simulink model "MAS_FTESO"  (R2022b)
settings: Solver=ode4  StartTime=0.0  StopTime=30  FixedStep=0.01  RelTol=1e-3
(part 2 of 3)

== matlab function MAS_FTESO/Control and plant 5/LP-based controller/Linear programming optimisation ==
  data: u_nom input; u_i output; G_i input; now output; expect output; expect input
function [u_i, now, expect] = linear_programming(u_nom, G_i, expect)

%% This function performs the optimisation via linear programming
% Input:
% u_ei: The nominal sliding mode control input for error reduction
% u_mi: The nominal sliding mode control input for acceleration tracking
% G_i: The control gain matrix
% Output:
% u_i: The optimised control input
% expect: The expected control performance

%% Find out the constrains
U_M = 0.2;

% Saturate the maintain control input
% u_mi_max = U_M;
% u_mi = min( u_mi_max * ones(size(u_mi)) , max(u_mi , - u_mi_max * ones(size(u_mi))) );

flag = 0;
u_i = u_nom;
for i = 1 : size(u_i,1)
    if abs(u_i(i))>U_M
        flag = 1;   % flag turns 1 if the limit is reached
        break;
    end
end

% Call the linear programming solver from MATLAB
coder.extrinsic('linprog');

if flag == 1
    
    %% Intialisation
    % Restrictions on inequalities
    A_ine = zeros(2*size(u_nom,1), size(u_nom,1));
    b_ine = zeros(2*size(u_nom,1), 1);
    num_ine = 0;
    
    % Restrictions on qualities
    A_equ = zeros(2*size(u_nom,1), size(u_nom,1));
    b_equ = zeros(2*size(u_nom,1), 1);
    num_equ = 0;
    
    %% Upper and lower bound from saturation
    lb = - U_M * ones(size(u_nom));
    ub = U_M * ones(size(u_nom));
    
    %% Restrictions according to expect
    for i = 1 : size(u_nom,1)
        if expect(i) == 0 % leading to equalities
            num_equ = num_equ + 1;
            A_equ(num_equ, :) = G_i(i,:);
        else
            % No extra effort
            num_ine = num_ine + 1;
            A_ine(num_ine,:) = sign(expect(i)) * G_i(i,:);
            b_ine(num_ine) = abs(expect(i));
            
            % Avoid inverse effect (same sign)
            num_ine = num_ine + 1;
            A_ine(num_ine,:) = - sign(expect(i)) * G_i(i,:);
            
        end
    end
    
    %% Restriction to keep the same direction   
       
    % Average cost function
    F_4 = -G_i(1,:) * sign(expect(1)) - G_i(2,:) * sign(expect(2)) - G_i(3,:) * sign(expect(3));
    
    F_5 = -G_i(1,:) * expect(1) - G_i(2,:) * expect(2) - G_i(3,:) * expect(3);
    
    F=F_4;

    u_i = linprog(F,A_ine(1:num_ine,:),b_ine(1:num_ine), A_equ(1:num_equ,:), b_equ(1:num_equ),lb,ub);
end

now = G_i * u_i;

end

== matlab function MAS_FTESO/Control and plant 4/Information subtracting ==
  data: e_xi output; L input; info_commu input; info_control input; delta_xi output; delta_vi output; a_di output; u_i_hat output; s_i output
function [e_xi, delta_xi, delta_vi, a_di, u_i_hat, s_i]=info_subtracting(L, info_commu,info_control)

%% This function is built to subtract the useful information for the controller design

% info_commu is in the format of [x_1,v_1,....,x_N,v_N]
% info_control is in the format of [delta_xi, delta_vi, a_di, w_i_hat]

serial_num = 4;
dimension = 3;
lambda = 2;

% For multiple system, we first seperate info_commu into delta_xi and delta_vi
num_agent = size(L,1);

delta_x = kron( kron(eye(num_agent) , [1,0] ), eye(dimension) ) * info_commu;
delta_v = kron( kron(eye(num_agent) , [0,1] ), eye(dimension) ) * info_commu;

L_i = kron( L(serial_num,:), eye(dimension) );
    
% Local errors calculating
e_xi = L_i * delta_x;
e_vi = L_i * delta_v;

% Substracting info_control
delta_xi = info_control(dimension*0+1:dimension*1);
delta_vi = info_control(dimension*1+1:dimension*2);

a_di = info_control(dimension*2+1:dimension*3);
u_i_hat = info_control(dimension*3+1:dimension*4);

% Slide variable
s_i = lambda * e_xi + e_vi;

end

== matlab function MAS_FTESO/Control and plant 4/LP-based controller/Linear programming optimisation ==
  data: u_nom input; u_i output; G_i input; now output; expect output; expect input
function [u_i, now, expect] = linear_programming(u_nom, G_i, expect)

%% This function performs the optimisation via linear programming
% Input:
% u_ei: The nominal sliding mode control input for error reduction
% u_mi: The nominal sliding mode control input for acceleration tracking
% G_i: The control gain matrix
% Output:
% u_i: The optimised control input
% expect: The expected control performance

%% Find out the constrains
U_M = 0.2;

% Saturate the maintain control input
% u_mi_max = U_M;
% u_mi = min( u_mi_max * ones(size(u_mi)) , max(u_mi , - u_mi_max * ones(size(u_mi))) );

flag = 0;
u_i = u_nom;
for i = 1 : size(u_i,1)
    if abs(u_i(i))>U_M
        flag = 1;   % flag turns 1 if the limit is reached
        break;
    end
end

% Call the linear programming solver from MATLAB
coder.extrinsic('linprog');

if flag == 1
    
    %% Intialisation
    % Restrictions on inequalities
    A_ine = zeros(2*size(u_nom,1), size(u_nom,1));
    b_ine = zeros(2*size(u_nom,1), 1);
    num_ine = 0;
    
    % Restrictions on qualities
    A_equ = zeros(2*size(u_nom,1), size(u_nom,1));
    b_equ = zeros(2*size(u_nom,1), 1);
    num_equ = 0;
    
    %% Upper and lower bound from saturation
    lb = - U_M * ones(size(u_nom));
    ub = U_M * ones(size(u_nom));
    
    %% Restrictions according to expect
    for i = 1 : size(u_nom,1)
        if expect(i) == 0 % leading to equalities
            num_equ = num_equ + 1;
            A_equ(num_equ, :) = G_i(i,:);
        else
            % No extra effort
            num_ine = num_ine + 1;
            A_ine(num_ine,:) = sign(expect(i)) * G_i(i,:);
            b_ine(num_ine) = abs(expect(i));
            
            % Avoid inverse effect (same sign)
            num_ine = num_ine + 1;
            A_ine(num_ine,:) = - sign(expect(i)) * G_i(i,:);
            
        end
    end
    
    %% Restriction to keep the same direction   
       
    % Average cost function
    F_4 = -G_i(1,:) * sign(expect(1)) - G_i(2,:) * sign(expect(2)) - G_i(3,:) * sign(expect(3));
    
    F_5 = -G_i(1,:) * expect(1) - G_i(2,:) * expect(2) - G_i(3,:) * expect(3);
    
    F=F_4;

    u_i = linprog(F,A_ine(1:num_ine,:),b_ine(1:num_ine), A_equ(1:num_equ,:), b_equ(1:num_equ),lb,ub);
end

now = G_i * u_i;

end

== matlab function MAS_FTESO/Control and plant 3/Information subtracting ==
  data: e_xi output; L input; info_commu input; info_control input; delta_xi output; delta_vi output; a_di output; u_i_hat output; s_i output
function [e_xi, delta_xi, delta_vi, a_di, u_i_hat, s_i]=info_subtracting(L, info_commu,info_control)

%% This function is built to subtract the useful information for the controller design

% info_commu is in the format of [x_1,v_1,....,x_N,v_N]
% info_control is in the format of [delta_xi, delta_vi, a_di, w_i_hat]

serial_num = 3;
dimension = 3;
lambda = 2;

% For multiple system, we first seperate info_commu into delta_xi and delta_vi
num_agent = size(L,1);

delta_x = kron( kron(eye(num_agent) , [1,0] ), eye(dimension) ) * info_commu;
delta_v = kron( kron(eye(num_agent) , [0,1] ), eye(dimension) ) * info_commu;

L_i = kron( L(serial_num,:), eye(dimension) );
    
% Local errors calculating
e_xi = L_i * delta_x;
e_vi = L_i * delta_v;

% Substracting info_control
delta_xi = info_control(dimension*0+1:dimension*1);
delta_vi = info_control(dimension*1+1:dimension*2);

a_di = info_control(dimension*2+1:dimension*3);
u_i_hat = info_control(dimension*3+1:dimension*4);

% Slide variable
s_i = lambda * e_xi + e_vi;

end

== matlab function MAS_FTESO/Self-calculation 3/Observer/Estimation sliding surface ==
  data: state input; state_hat input; esti_x output
function esti_x   = esti_slide(state,state_hat)

%% This function represents the self-iteration of the observer itself
dimension = 3;

% Seperate the state information
x = state(dimension*0+1:dimension*1);

% Seperate the state estiamtion
x_hat = state_hat(dimension*0+1:dimension*1);

% Estimation error vectors
esti_x = x - x_hat;

end

== matlab function MAS_FTESO/Control and plant 3/LP-based controller/Linear programming optimisation ==
  data: u_nom input; u_i output; G_i input; now output; expect output; expect input
function [u_i, now, expect] = linear_programming(u_nom, G_i, expect)

%% This function performs the optimisation via linear programming
% Input:
% u_ei: The nominal sliding mode control input for error reduction
% u_mi: The nominal sliding mode control input for acceleration tracking
% G_i: The control gain matrix
% Output:
% u_i: The optimised control input
% expect: The expected control performance

%% Find out the constrains
U_M = 0.2;

% Saturate the maintain control input
% u_mi_max = U_M;
% u_mi = min( u_mi_max * ones(size(u_mi)) , max(u_mi , - u_mi_max * ones(size(u_mi))) );

flag = 0;
u_i = u_nom;
for i = 1 : size(u_i,1)
    if abs(u_i(i))>U_M
        flag = 1;   % flag turns 1 if the limit is reached
        break;
    end
end

% Call the linear programming solver from MATLAB
coder.extrinsic('linprog');

if flag == 1
    
    %% Intialisation
    % Restrictions on inequalities
    A_ine = zeros(2*size(u_nom,1), size(u_nom,1));
    b_ine = zeros(2*size(u_nom,1), 1);
    num_ine = 0;
    
    % Restrictions on qualities
    A_equ = zeros(2*size(u_nom,1), size(u_nom,1));
    b_equ = zeros(2*size(u_nom,1), 1);
    num_equ = 0;
    
    %% Upper and lower bound from saturation
    lb = - U_M * ones(size(u_nom));
    ub = U_M * ones(size(u_nom));
    
    %% Restrictions according to expect
    for i = 1 : size(u_nom,1)
        if expect(i) == 0 % leading to equalities
            num_equ = num_equ + 1;
            A_equ(num_equ, :) = G_i(i,:);
        else
            % No extra effort
            num_ine = num_ine + 1;
            A_ine(num_ine,:) = sign(expect(i)) * G_i(i,:);
            b_ine(num_ine) = abs(expect(i));
            
            % Avoid inverse effect (same sign)
            num_ine = num_ine + 1;
            A_ine(num_ine,:) = - sign(expect(i)) * G_i(i,:);
            
        end
    end
    
    %% Restriction to keep the same direction   
       
    % Average cost function
    F_4 = -G_i(1,:) * sign(expect(1)) - G_i(2,:) * sign(expect(2)) - G_i(3,:) * sign(expect(3));
    
    F_5 = -G_i(1,:) * expect(1) - G_i(2,:) * expect(2) - G_i(3,:) * expect(3);
    
    F=F_4;

    u_i = linprog(F,A_ine(1:num_ine,:),b_ine(1:num_ine), A_equ(1:num_equ,:), b_equ(1:num_equ),lb,ub);
end

now = G_i * u_i;

end

== matlab function MAS_FTESO/Control and plant 1/LP-based controller/Nominal Controller ==
  data: x_i input; u_i output; delta_xi input; delta_vi input; a_di input; u_i_hat input; s_i input; xi_i input; G_i output; expect output
function [u_i, G_i, expect] = fcn(x_i, delta_xi, delta_vi, a_di, u_i_hat, s_i, xi_i)

%% This is the controller design for each agent
%% Controller parameters
c_i = 2;
lambda_i = 2;

%% Basic model parameters
Radius = [0.20,0.22,0.21,0.19,0.23,0.18];   

%% The parameter of individual agent
serial_num = 1; 
R=Radius(serial_num);

%% Robot orientation
theta = x_i(3);

%% Input coupling matrix
G_i=[-sin(theta), -sin(pi/3-theta), sin(pi/3+theta);
    cos(theta), -cos(pi/3-theta), -cos(pi/3+theta);
    1/R,          1/R,                  1/R];

%% Nominal control input
expect = a_di - u_i_hat - lambda_i * delta_vi - c_i * s_i - delta_xi - c_i * xi_i;
u_i = G_i^(-1) * expect;

end

== matlab function MAS_FTESO/Control and plant 3/LP-based controller/Nominal Controller ==
  data: x_i input; u_i output; delta_xi input; delta_vi input; a_di input; u_i_hat input; s_i input; xi_i input; G_i output; expect output
function [u_i, G_i, expect] = fcn(x_i, delta_xi, delta_vi, a_di, u_i_hat, s_i, xi_i)

%% This is the controller design for each agent
%% Controller parameters
c_i = 2;
lambda_i = 2;

%% Basic model parameters
Radius = [0.20,0.22,0.21,0.19,0.23,0.18];   

%% The parameter of individual agent
serial_num = 3; 
R=Radius(serial_num);

%% Robot orientation
theta = x_i(3);

%% Input coupling matrix
G_i=[-sin(theta), -sin(pi/3-theta), sin(pi/3+theta);
    cos(theta), -cos(pi/3-theta), -cos(pi/3+theta);
    1/R,          1/R,                  1/R];

%% Nominal control input
expect = a_di - u_i_hat - lambda_i * delta_vi - c_i * s_i - delta_xi - c_i * xi_i;
u_i = G_i^(-1) * expect;

end

== matlab function MAS_FTESO/Self-calculation 1/Observer/Estimation sliding surface ==
  data: state input; state_hat input; esti_x output
function esti_x   = esti_slide(state,state_hat)

%% This function represents the self-iteration of the observer itself
dimension = 3;

% Seperate the state information
x = state(dimension*0+1:dimension*1);

% Seperate the state estiamtion
x_hat = state_hat(dimension*0+1:dimension*1);

% Estimation error vectors
esti_x = x - x_hat;

end

== matlab function MAS_FTESO/Self-calculation 1/Observer/MATLAB Function ==
  data: state_hat input; w_i_hat output
function w_i_hat = fcn(state_hat)

dimension = 3;

w_i_hat = state_hat(dimension * 2 + 1 : dimension * 3);

end

== matlab function MAS_FTESO/Self-calculation 2/Observer/Estimation sliding surface ==
  data: state input; state_hat input; esti_x output
function esti_x   = esti_slide(state,state_hat)

%% This function represents the self-iteration of the observer itself
dimension = 3;

% Seperate the state information
x = state(dimension*0+1:dimension*1);

% Seperate the state estiamtion
x_hat = state_hat(dimension*0+1:dimension*1);

% Estimation error vectors
esti_x = x - x_hat;

end

== matlab function MAS_FTESO/Self-calculation 2/Observer/MATLAB Function ==
  data: state_hat input; w_i_hat output
function w_i_hat = fcn(state_hat)

dimension = 3;

w_i_hat = state_hat(dimension * 2 + 1 : dimension * 3);

end

== matlab function MAS_FTESO/Self-calculation 1/Observer/Observer iteration ==
  data: state_hat_dot output; state input; u_i input; x_tilde input; state_hat input
function state_hat_dot  = eso(state, u_i, x_tilde, state_hat)

serial_num = 1;
dimension = 3;
Radius = [0.20,0.22,0.21,0.19,0.23,0.18];
R = Radius(serial_num);
theta = state(dimension);
g=[-sin(theta), -sin(pi/3-theta), sin(pi/3+theta);
    cos(theta), -cos(pi/3-theta), -cos(pi/3+theta);
    1/R,          1/R,                  1/R];

alpha_1 = 4/5;
alpha_2 = 3/5;
beta_1 = 5 * eye(3);
beta_2 = 10 * eye(3);
beta_3 = 100 * eye(3);
rho = 2 * eye(3);

x_hat_dot = state_hat(dimension * 1 + 1 : dimension * 2) + beta_1 * (diag(sign(x_tilde)) * abs(x_tilde).^alpha_1 + x_tilde );
v_hat_dot = state_hat(dimension * 2 + 1 : dimension * 3) + beta_2 * (diag(sign(x_tilde)) * abs(x_tilde).^alpha_2 + rho * x_tilde ) + g * u_i;
w_hat_dot = beta_3 * ( diag(sign(x_tilde)) * abs(x_tilde).^alpha_2 + rho * x_tilde );

state_hat_dot = [x_hat_dot; v_hat_dot; w_hat_dot]; 

end

== matlab function MAS_FTESO/Self-calculation 3/Observer/MATLAB Function ==
  data: state_hat input; w_i_hat output
function w_i_hat = fcn(state_hat)

dimension = 3;

w_i_hat = state_hat(dimension * 2 + 1 : dimension * 3);

end

== matlab function MAS_FTESO/Control and plant 1/System Plant1 ==
  settings: updateMethod=DISCRETE
  data: agent_x input; v_dot output; agent_v input; t input; control_input input; w output
function [v_dot, w] = physical_model( agent_x , agent_v, t, control_input )

%% Note
% System output
% v_dot: the acceleration vector
% w: the matched disturbances
% saturation status: off
% model is established by the driving force provided by the motor

%% basic parameters set of agents
Mass = [3,3.2,2.8,2.6,3.1,2.9];
Radius = [0.20,0.22,0.21,0.19,0.23,0.18];
Inertia = [0.08,0.10,0.07,0.05,0.09,0.06];

%% assign the parameter according to serial number
serial_num = 1; 
m=Mass(serial_num);
R=Radius(serial_num);
inertia=Inertia(serial_num);

%% current states of the robot
dimension=3;

x=agent_x(1);
y=agent_x(2);
theta=agent_x(dimension);

%% time-varying matched disturbances
% matched_disturbance= [0.5*sin(1.5*t+pi/4*serial_num+x)+2; 0.6*cos(2*t+pi/3*serial_num+0.5*y)+1.5; 0.5*sin(0.8*t+pi/5*serial_num+0.4*theta)+1];

% matched_disturbance= [0.5*sin(1.5*t+pi/4*serial_num)+2; 0.6*cos(2*t+pi/3*serial_num)+1.5; 0.5*sin(0.8*t+pi/5*serial_num)+1];
matched_disturbance = 0.2 * [0.5*sin(x) + 0.5*sin(0.6*t + pi/5*serial_num); - 0.6*exp(-abs(y)-1) + 0.4*sin(0.4*t + pi/5*serial_num) ; 0.2 * cos(theta) + 0.3 * sin(0.5*t + pi/5*serial_num)];
% matched_disturbance = matched_disturbance + noise;
%% the real model of robot
M=diag([1/m,1/m,1/inertia]);
g=[-sin(theta), -sin(pi/3-theta), sin(pi/3+theta);
    cos(theta), -cos(pi/3-theta), -cos(pi/3+theta);
    1/R,          1/R,                  1/R];


%% plant output

w = matched_disturbance;

v_dot = w + g* control_input;


end

== matlab function MAS_FTESO/Control and plant 4/LP-based controller/Nominal Controller ==
  data: x_i input; u_i output; delta_xi input; delta_vi input; a_di input; u_i_hat input; s_i input; xi_i input; G_i output; expect output
function [u_i, G_i, expect] = fcn(x_i, delta_xi, delta_vi, a_di, u_i_hat, s_i, xi_i)

%% This is the controller design for each agent
%% Controller parameters
c_i = 2;
lambda_i = 2;

%% Basic model parameters
Radius = [0.20,0.22,0.21,0.19,0.23,0.18];   

%% The parameter of individual agent
serial_num = 4; 
R=Radius(serial_num);

%% Robot orientation
theta = x_i(3);

%% Input coupling matrix
G_i=[-sin(theta), -sin(pi/3-theta), sin(pi/3+theta);
    cos(theta), -cos(pi/3-theta), -cos(pi/3+theta);
    1/R,          1/R,                  1/R];

%% Nominal control input
expect = a_di - u_i_hat - lambda_i * delta_vi - c_i * s_i - delta_xi - c_i * xi_i;
u_i = G_i^(-1) * expect;

end

== matlab function MAS_FTESO/Control and plant 5/LP-based controller/Nominal Controller ==
  data: x_i input; u_i output; delta_xi input; delta_vi input; a_di input; u_i_hat input; s_i input; xi_i input; G_i output; expect output
function [u_i, G_i, expect] = fcn(x_i, delta_xi, delta_vi, a_di, u_i_hat, s_i, xi_i)

%% This is the controller design for each agent
%% Controller parameters
c_i = 2;
lambda_i = 2;

%% Basic model parameters
Radius = [0.20,0.22,0.21,0.19,0.23,0.18];   

%% The parameter of individual agent
serial_num = 5; 
R=Radius(serial_num);

%% Robot orientation
theta = x_i(3);

%% Input coupling matrix
G_i=[-sin(theta), -sin(pi/3-theta), sin(pi/3+theta);
    cos(theta), -cos(pi/3-theta), -cos(pi/3+theta);
    1/R,          1/R,                  1/R];

%% Nominal control input
expect = a_di - u_i_hat - lambda_i * delta_vi - c_i * s_i - delta_xi - c_i * xi_i;
u_i = G_i^(-1) * expect;

end

== matlab function MAS_FTESO/Control and plant 6/LP-based controller/Nominal Controller ==
  data: x_i input; u_i output; delta_xi input; delta_vi input; a_di input; u_i_hat input; s_i input; xi_i input; G_i output; expect output
function [u_i, G_i, expect] = fcn(x_i, delta_xi, delta_vi, a_di, u_i_hat, s_i, xi_i)

%% This is the controller design for each agent
%% Controller parameters
c_i = 2;
lambda_i = 2;

%% Basic model parameters
Radius = [0.20,0.22,0.21,0.19,0.23,0.18];   

%% The parameter of individual agent
serial_num = 6; 
R=Radius(serial_num);

%% Robot orientation
theta = x_i(3);

%% Input coupling matrix
G_i=[-sin(theta), -sin(pi/3-theta), sin(pi/3+theta);
    cos(theta), -cos(pi/3-theta), -cos(pi/3+theta);
    1/R,          1/R,                  1/R];

%% Nominal control input
expect = a_di - u_i_hat - lambda_i * delta_vi - c_i * s_i - delta_xi - c_i * xi_i;
u_i = G_i^(-1) * expect;

end

== matlab function MAS_FTESO/Control and plant 1/LP-based controller/Subsystem/Auxiliary variable ==
  data: G_i input; u_tilde input; xi_dot output; xi_prev input
function xi_dot = aux_updata(G_i, u_tilde, xi_prev)

eta_4 = diag([3,3,2]);
eta_5 = diag([0.5,0.5,0.5]);

if norm(xi_prev) >= 10
    xi_dot = eta_4 * G_i * u_tilde - eta_5 * xi_prev;
else
    xi_dot = eta_4 * G_i * u_tilde - eta_5 * xi_prev - norm(u_tilde)^2/norm(xi_prev)^2 * xi_prev;
end

end

== matlab function MAS_FTESO/Self-calculation 4/Observer/Estimation sliding surface ==
  data: state input; state_hat input; esti_x output
function esti_x   = esti_slide(state,state_hat)

%% This function represents the self-iteration of the observer itself
dimension = 3;

% Seperate the state information
x = state(dimension*0+1:dimension*1);

% Seperate the state estiamtion
x_hat = state_hat(dimension*0+1:dimension*1);

% Estimation error vectors
esti_x = x - x_hat;

end

== matlab function MAS_FTESO/Self-calculation 3/Observer/Observer iteration ==
  data: state_hat_dot output; state input; u_i input; x_tilde input; state_hat input
function state_hat_dot  = eso(state, u_i, x_tilde, state_hat)

serial_num = 3;
dimension = 3;
Radius = [0.20,0.22,0.21,0.19,0.23,0.18];
R = Radius(serial_num);
theta = state(dimension);
g=[-sin(theta), -sin(pi/3-theta), sin(pi/3+theta);
    cos(theta), -cos(pi/3-theta), -cos(pi/3+theta);
    1/R,          1/R,                  1/R];

alpha_1 = 4/5;
alpha_2 = 3/5;
beta_1 = 5 * eye(3);
beta_2 = 10 * eye(3);
beta_3 = 100 * eye(3);
rho = 2 * eye(3);

x_hat_dot = state_hat(dimension * 1 + 1 : dimension * 2) + beta_1 * (diag(sign(x_tilde)) * abs(x_tilde).^alpha_1 + x_tilde );
v_hat_dot = state_hat(dimension * 2 + 1 : dimension * 3) + beta_2 * (diag(sign(x_tilde)) * abs(x_tilde).^alpha_2 + rho * x_tilde ) + g * u_i;
w_hat_dot = beta_3 * ( diag(sign(x_tilde)) * abs(x_tilde).^alpha_2 + rho * x_tilde );

state_hat_dot = [x_hat_dot; v_hat_dot; w_hat_dot]; 

end

== matlab function MAS_FTESO/Self-calculation 4/Observer/MATLAB Function ==
  data: state_hat input; w_i_hat output
function w_i_hat = fcn(state_hat)

dimension = 3;

w_i_hat = state_hat(dimension * 2 + 1 : dimension * 3);

end

== matlab function MAS_FTESO/Control and plant 3/LP-based controller/Subsystem/Auxiliary variable ==
  data: G_i input; u_tilde input; xi_dot output; xi_prev input
function xi_dot = aux_updata(G_i, u_tilde, xi_prev)

eta_4 = diag([3,3,2]);
eta_5 = diag([0.5,0.5,0.5]);

if norm(xi_prev) >= 10
    xi_dot = eta_4 * G_i * u_tilde - eta_5 * xi_prev;
else
    xi_dot = eta_4 * G_i * u_tilde - eta_5 * xi_prev - norm(u_tilde)^2/norm(xi_prev)^2 * xi_prev;
end

end

== matlab function MAS_FTESO/Self-calculation 4/Observer/Observer iteration ==
  data: state_hat_dot output; state input; u_i input; x_tilde input; state_hat input
function state_hat_dot  = eso(state, u_i, x_tilde, state_hat)

serial_num = 4;
dimension = 3;
Radius = [0.20,0.22,0.21,0.19,0.23,0.18];
R = Radius(serial_num);
theta = state(dimension);
g=[-sin(theta), -sin(pi/3-theta), sin(pi/3+theta);
    cos(theta), -cos(pi/3-theta), -cos(pi/3+theta);
    1/R,          1/R,                  1/R];

alpha_1 = 4/5;
alpha_2 = 3/5;
beta_1 = 5 * eye(3);
beta_2 = 10 * eye(3);
beta_3 = 100 * eye(3);
rho = 2 * eye(3);

x_hat_dot = state_hat(dimension * 1 + 1 : dimension * 2) + beta_1 * (diag(sign(x_tilde)) * abs(x_tilde).^alpha_1 + x_tilde );
v_hat_dot = state_hat(dimension * 2 + 1 : dimension * 3) + beta_2 * (diag(sign(x_tilde)) * abs(x_tilde).^alpha_2 + rho * x_tilde ) + g * u_i;
w_hat_dot = beta_3 * ( diag(sign(x_tilde)) * abs(x_tilde).^alpha_2 + rho * x_tilde );

state_hat_dot = [x_hat_dot; v_hat_dot; w_hat_dot]; 

end

== matlab function MAS_FTESO/Control and plant 4/LP-based controller/Subsystem/Auxiliary variable ==
  data: G_i input; u_tilde input; xi_dot output; xi_prev input
function xi_dot = aux_updata(G_i, u_tilde, xi_prev)

eta_4 = diag([3,3,2]);
eta_5 = diag([0.5,0.5,0.5]);

if norm(xi_prev) >= 10
    xi_dot = eta_4 * G_i * u_tilde - eta_5 * xi_prev;
else
    xi_dot = eta_4 * G_i * u_tilde - eta_5 * xi_prev - norm(u_tilde)^2/norm(xi_prev)^2 * xi_prev;
end

end

== matlab function MAS_FTESO/Control and plant 5/LP-based controller/Subsystem/Auxiliary variable ==
  data: G_i input; u_tilde input; xi_dot output; xi_prev input
function xi_dot = aux_updata(G_i, u_tilde, xi_prev)

eta_4 = diag([3,3,2]);
eta_5 = diag([0.5,0.5,0.5]);

if norm(xi_prev) >= 10
    xi_dot = eta_4 * G_i * u_tilde - eta_5 * xi_prev;
else
    xi_dot = eta_4 * G_i * u_tilde - eta_5 * xi_prev - norm(u_tilde)^2/norm(xi_prev)^2 * xi_prev;
end

end

== matlab function MAS_FTESO/Control and plant 6/LP-based controller/Subsystem/Auxiliary variable ==
  data: G_i input; u_tilde input; xi_dot output; xi_prev input
function xi_dot = aux_updata(G_i, u_tilde, xi_prev)

eta_4 = diag([3,3,2]);
eta_5 = diag([0.5,0.5,0.5]);

if norm(xi_prev) >= 10
    xi_dot = eta_4 * G_i * u_tilde - eta_5 * xi_prev;
else
    xi_dot = eta_4 * G_i * u_tilde - eta_5 * xi_prev - norm(u_tilde)^2/norm(xi_prev)^2 * xi_prev;
end

end

== matlab function MAS_FTESO/Self-calculation 5/Observer1/Estimation sliding surface ==
  data: state input; state_hat input; esti_x output
function esti_x   = esti_slide(state,state_hat)

%% This function represents the self-iteration of the observer itself
dimension = 3;

% Seperate the state information
x = state(dimension*0+1:dimension*1);

% Seperate the state estiamtion
x_hat = state_hat(dimension*0+1:dimension*1);

% Estimation error vectors
esti_x = x - x_hat;

end

== matlab function MAS_FTESO/Self-calculation 5/Observer1/MATLAB Function ==
  data: state_hat input; w_i_hat output
function w_i_hat = fcn(state_hat)

dimension = 3;

w_i_hat = state_hat(dimension * 2 + 1 : dimension * 3);

end

== matlab function MAS_FTESO/Self-calculation 5/Observer1/Observer iteration ==
  data: state_hat_dot output; state input; u_i input; x_tilde input; state_hat input
function state_hat_dot  = eso(state, u_i, x_tilde, state_hat)

serial_num = 5;
dimension = 3;
Radius = [0.20,0.22,0.21,0.19,0.23,0.18];
R = Radius(serial_num);
theta = state(dimension);
g=[-sin(theta), -sin(pi/3-theta), sin(pi/3+theta);
    cos(theta), -cos(pi/3-theta), -cos(pi/3+theta);
    1/R,          1/R,                  1/R];

alpha_1 = 4/5;
alpha_2 = 3/5;
beta_1 = 5 * eye(3);
beta_2 = 10 * eye(3);
beta_3 = 100 * eye(3);
rho = 2 * eye(3);

x_hat_dot = state_hat(dimension * 1 + 1 : dimension * 2) + beta_1 * (diag(sign(x_tilde)) * abs(x_tilde).^alpha_1 + x_tilde );
v_hat_dot = state_hat(dimension * 2 + 1 : dimension * 3) + beta_2 * (diag(sign(x_tilde)) * abs(x_tilde).^alpha_2 + rho * x_tilde ) + g * u_i;
w_hat_dot = beta_3 * ( diag(sign(x_tilde)) * abs(x_tilde).^alpha_2 + rho * x_tilde );

state_hat_dot = [x_hat_dot; v_hat_dot; w_hat_dot]; 

end

== matlab function MAS_FTESO/Self-calculation 6/Observer1/Estimation sliding surface ==
  data: state input; state_hat input; esti_x output
function esti_x   = esti_slide(state,state_hat)

%% This function represents the self-iteration of the observer itself
dimension = 3;

% Seperate the state information
x = state(dimension*0+1:dimension*1);

% Seperate the state estiamtion
x_hat = state_hat(dimension*0+1:dimension*1);

% Estimation error vectors
esti_x = x - x_hat;

end

== matlab function MAS_FTESO/Reference Generator/Acceleration Reference ==
  data: t input; a_d output; centre output
function [a_d, centre] = gene_ref_x1(t)

%% Generate acceleration reference
% This function can generate the reference trajectory for a rotating
% rectangular

%% Formation centre (the centre of the rectangular)
% centre of the formation reference (circular moving trajectory)
R_c = 1;
w_c = -0.1;
x_c = -w_c^2 * R_c * cos(w_c * t);
y_c = -w_c^2 * R_c * sin(w_c * t);
centre = [x_c; y_c]; 
% Parameters for the circular trajectory
R = 2;
w = 0.1;
x1 = [x_c - R * w^2 * cos( w * t + 1/3 * pi); y_c - R * w^2 * sin( w * t + 1/3 * pi); 0];
x2 = [x_c - R * w^2 * cos( w * t + 2/3 * pi); y_c - R * w^2 * sin( w * t + 2/3 * pi); 0];
x3 = [x_c - R * w^2 * cos( w * t + 3/3 * pi); y_c - R * w^2 * sin( w * t + 3/3 * pi); 0];
x4 = [x_c - R * w^2 * cos( w * t + 4/3 * pi); y_c - R * w^2 * sin( w * t + 4/3 * pi); 0];
x5 = [x_c - R * w^2 * cos( w * t + 5/3 * pi); y_c - R * w^2 * sin( w * t + 5/3 * pi); 0];
x6 = [x_c - R * w^2 * cos( w * t + 6/3 * pi); y_c - R * w^2 * sin( w * t + 6/3 * pi); 0];

a_d=[x1;x2;x3;x4;x5;x6];


end

== matlab function MAS_FTESO/Self-calculation 1/Tracking error calculation/Data selection ==
  data: ref input; delta_xi output; state input; delta_vi output; a_d output
function [delta_xi, delta_vi, a_d] = data_selection(ref, state)

%% This function is built to select the reference information and obtain the tracking error
serial_num = 1; 
dimension = 3;
num_agent = 6;

% Seperate the reference vector
pos_ref = ref(dimension*num_agent * 0 + 1 : dimension*num_agent * 1);
vel_ref = ref(dimension*num_agent * 1 + 1 : dimension*num_agent * 2);
acc_ref = ref(dimension*num_agent * 2 + 1 : dimension*num_agent * 3);

% Find out the reference for the current agent
pos_d = pos_ref( (serial_num-1) * dimension + 1 : serial_num * dimension);
vel_d = vel_ref( (serial_num-1) * dimension + 1 : serial_num * dimension);
acc_d = acc_ref( (serial_num-1) * dimension + 1 : serial_num * dimension);

% Seperate the state vector
x_i = state(dimension*0+1:dimension*1);
v_i = state(dimension*1+1:dimension*2);

% Calculate the error
delta_xi = x_i - pos_d;
delta_vi = v_i - vel_d;
a_d = acc_d;


end

== matlab function MAS_FTESO/Reference Generator/Position Reference ==
  data: t input; x_d output; centre output
function [x_d, centre] = gene_ref_x1(t)

%% Generate position reference
% This function can generate the reference trajectory for a rotating
% rectangular

%% Formation centre (the centre of the rectangular)
% centre of the formation reference (circular moving trajectory)
R_c = 1;
w_c = -0.1;
x_c = R_c * cos(w_c * t);
y_c = R_c * sin(w_c * t);
centre = [x_c; y_c]; 
% Parameters for the circular trajectory
R = 2;
w = 0.1;
x1 = [x_c + R * cos( w * t + 1/3 * pi); y_c + R * sin( w * t + 1/3 * pi); 0];
x2 = [x_c + R * cos( w * t + 2/3 * pi); y_c + R * sin( w * t + 2/3 * pi); 0];
x3 = [x_c + R * cos( w * t + 3/3 * pi); y_c + R * sin( w * t + 3/3 * pi); 0];
x4 = [x_c + R * cos( w * t + 4/3 * pi); y_c + R * sin( w * t + 4/3 * pi); 0];
x5 = [x_c + R * cos( w * t + 5/3 * pi); y_c + R * sin( w * t + 5/3 * pi); 0];
x6 = [x_c + R * cos( w * t + 6/3 * pi); y_c + R * sin( w * t + 6/3 * pi); 0];

x_d=[x1;x2;x3;x4;x5;x6];


end

== matlab function MAS_FTESO/Reference Generator/Velocity Reference ==
  data: t input; v_d output; centre output
function [v_d, centre] = gene_ref_x2(t)

%% Generate velocity reference
% This function can generate the reference trajectory for a rotating
% rectangular

%% Formation centre (the centre of the rectangular)
% centre of the formation reference (circular moving trajectory)
R_c = 1;
w_c = -0.1;
x_c = -w_c * R_c * sin(w_c * t);
y_c =  w_c * R_c * cos(w_c * t);
centre = [x_c; y_c]; 
% Parameters for the circular trajectory
R = 2;
w = 0.1;
x1 = [x_c - R * w * sin( w * t + 1/3 * pi); y_c + R * w * cos( w * t + 1/3 * pi); 0];
x2 = [x_c - R * w * sin( w * t + 2/3 * pi); y_c + R * w * cos( w * t + 2/3 * pi); 0];
x3 = [x_c - R * w * sin( w * t + 3/3 * pi); y_c + R * w * cos( w * t + 3/3 * pi); 0];
x4 = [x_c - R * w * sin( w * t + 4/3 * pi); y_c + R * w * cos( w * t + 4/3 * pi); 0];
x5 = [x_c - R * w * sin( w * t + 5/3 * pi); y_c + R * w * cos( w * t + 5/3 * pi); 0];
x6 = [x_c - R * w * sin( w * t + 6/3 * pi); y_c + R * w * cos( w * t + 6/3 * pi); 0];

v_d=[x1;x2;x3;x4;x5;x6];


end

== matlab function MAS_FTESO/Self-calculation 6/Observer1/MATLAB Function ==
  data: state_hat input; w_i_hat output
function w_i_hat = fcn(state_hat)

dimension = 3;

w_i_hat = state_hat(dimension * 2 + 1 : dimension * 3);

end

== matlab function MAS_FTESO/Control and plant 2/MATLAB Function ==
  data: u input; y output
function y = fcn(u)

y = norm(u);

end

== matlab function MAS_FTESO/Control and plant 2/System Plant1 ==
  settings: updateMethod=DISCRETE
  data: agent_x input; v_dot output; agent_v input; t input; control_input input; w output
function [v_dot, w] = physical_model( agent_x , agent_v, t, control_input )

%% Note
% System output
% v_dot: the acceleration vector
% w: the matched disturbances
% saturation status: off
% model is established by the driving force provided by the motor

%% basic parameters set of agents
Radius = [0.20,0.22,0.21,0.19,0.23,0.18];

%% assign the parameter according to serial number
serial_num = 2; 
R=Radius(serial_num);

%% current states of the robot
dimension=3;

x=agent_x(1);
y=agent_x(2);
theta=agent_x(dimension);

%% time-varying matched disturbances
% matched_disturbance= [0.5*sin(1.5*t+pi/4*serial_num+x)+2; 0.6*cos(2*t+pi/3*serial_num+0.5*y)+1.5; 0.5*sin(0.8*t+pi/5*serial_num+0.4*theta)+1];

% matched_disturbance= [0.5*sin(1.5*t+pi/4*serial_num)+2; 0.6*cos(2*t+pi/3*serial_num)+1.5; 0.5*sin(0.8*t+pi/5*serial_num)+1];
matched_disturbance = 0.2 * [0.5*sin(x) + 0.5*sin(0.6*t + pi/5*serial_num); - 0.6*exp(-abs(y)-1) + 0.4*sin(0.4*t + pi/5*serial_num) ; 0.2 * cos(theta) + 0.3 * sin(0.5*t + pi/5*serial_num)];
% matched_disturbance = matched_disturbance + noise;
%% the real model of robot
g=[-sin(theta), -sin(pi/3-theta), sin(pi/3+theta);
    cos(theta), -cos(pi/3-theta), -cos(pi/3+theta);
    1/R,          1/R,                  1/R];

%% plant output
w = matched_disturbance;

v_dot = w + g* control_input;


end

== matlab function MAS_FTESO/Control and plant 3/MATLAB Function ==
  data: u input; y output
function y = fcn(u)

y = norm(u);

end

== matlab function MAS_FTESO/Control and plant 3/System Plant1 ==
  settings: updateMethod=DISCRETE
  data: agent_x input; v_dot output; agent_v input; t input; control_input input; w output
function [v_dot, w] = physical_model( agent_x , agent_v, t, control_input )

%% Note
% System output
% v_dot: the acceleration vector
% w: the matched disturbances
% saturation status: off
% model is established by the driving force provided by the motor

%% basic parameters set of agents
Radius = [0.20,0.22,0.21,0.19,0.23,0.18];

%% assign the parameter according to serial number
serial_num = 3; 
R=Radius(serial_num);

%% current states of the robot
dimension=3;

x=agent_x(1);
y=agent_x(2);
theta=agent_x(dimension);

%% time-varying matched disturbances
% matched_disturbance= [0.5*sin(1.5*t+pi/4*serial_num+x)+2; 0.6*cos(2*t+pi/3*serial_num+0.5*y)+1.5; 0.5*sin(0.8*t+pi/5*serial_num+0.4*theta)+1];

% matched_disturbance= [0.5*sin(1.5*t+pi/4*serial_num)+2; 0.6*cos(2*t+pi/3*serial_num)+1.5; 0.5*sin(0.8*t+pi/5*serial_num)+1];
matched_disturbance = 0.2 * [0.5*sin(x) + 0.5*sin(0.6*t + pi/5*serial_num); - 0.6*exp(-abs(y)-1) + 0.4*sin(0.4*t + pi/5*serial_num) ; 0.2 * cos(theta) + 0.3 * sin(0.5*t + pi/5*serial_num)];
%% the real model of robot
g=[-sin(theta), -sin(pi/3-theta), sin(pi/3+theta);
    cos(theta), -cos(pi/3-theta), -cos(pi/3+theta);
    1/R,          1/R,                  1/R];

%% plant output
w = matched_disturbance;

v_dot = w + g* control_input;

end

== matlab function MAS_FTESO/Control and plant 4/MATLAB Function ==
  data: u input; y output
function y = fcn(u)

y = norm(u);

end

== matlab function MAS_FTESO/Control and plant 4/System Plant1 ==
  settings: updateMethod=DISCRETE
  data: agent_x input; v_dot output; agent_v input; t input; control_input input; w output
function [v_dot, w] = physical_model( agent_x , agent_v, t, control_input )

%% Note
% System output
% v_dot: the acceleration vector
% w: the matched disturbances
% saturation status: off
% model is established by the driving force provided by the motor

%% basic parameters set of agents
Radius = [0.20,0.22,0.21,0.19,0.23,0.18];

%% assign the parameter according to serial number
serial_num = 4; 
R=Radius(serial_num);

%% current states of the robot
dimension=3;

x=agent_x(1);
y=agent_x(2);
theta=agent_x(dimension);

%% time-varying matched disturbances
% matched_disturbance= [0.5*sin(1.5*t+pi/4*serial_num+x)+2; 0.6*cos(2*t+pi/3*serial_num+0.5*y)+1.5; 0.5*sin(0.8*t+pi/5*serial_num+0.4*theta)+1];

% matched_disturbance= [0.5*sin(1.5*t+pi/4*serial_num)+2; 0.6*cos(2*t+pi/3*serial_num)+1.5; 0.5*sin(0.8*t+pi/5*serial_num)+1];
matched_disturbance = 0.2 * [0.5*sin(x) + 0.5*sin(0.6*t + pi/5*serial_num); - 0.6*exp(-abs(y)-1) + 0.4*sin(0.4*t + pi/5*serial_num) ; 0.2 * cos(theta) + 0.3 * sin(0.5*t + pi/5*serial_num)];
%% the real model of robot
g=[-sin(theta), -sin(pi/3-theta), sin(pi/3+theta);
    cos(theta), -cos(pi/3-theta), -cos(pi/3+theta);
    1/R,          1/R,                  1/R];

%% plant output
w = matched_disturbance;

v_dot = w + g* control_input;


end

== matlab function MAS_FTESO/Control and plant 5/MATLAB Function ==
  data: u input; y output
function y = fcn(u)

y = norm(u);

end

== matlab function MAS_FTESO/Self-calculation 2/Tracking error calculation/Data selection ==
  data: ref input; delta_xi output; state input; delta_vi output; a_d output
function [delta_xi, delta_vi, a_d] = data_selection(ref, state)

%% This function is built to select the reference information and obtain the tracking error
serial_num = 2; 
dimension = 3;
num_agent = 6;

% Seperate the reference vector
pos_ref = ref(dimension*num_agent * 0 + 1 : dimension*num_agent * 1);
vel_ref = ref(dimension*num_agent * 1 + 1 : dimension*num_agent * 2);
acc_ref = ref(dimension*num_agent * 2 + 1 : dimension*num_agent * 3);

% Find out the reference for the current agent
pos_d = pos_ref( (serial_num-1) * dimension + 1 : serial_num * dimension);
vel_d = vel_ref( (serial_num-1) * dimension + 1 : serial_num * dimension);
acc_d = acc_ref( (serial_num-1) * dimension + 1 : serial_num * dimension);

% Seperate the state vector
x_i = state(dimension*0+1:dimension*1);
v_i = state(dimension*1+1:dimension*2);

% Calculate the error
delta_xi = x_i - pos_d;
delta_vi = v_i - vel_d;
a_d = acc_d;


end

== matlab function MAS_FTESO/Control and plant 5/System Plant1 ==
  settings: updateMethod=DISCRETE
  data: agent_x input; v_dot output; agent_v input; t input; control_input input; w output
function [v_dot, w] = physical_model( agent_x , agent_v, t, control_input )

%% Note
% System output
% v_dot: the acceleration vector
% w: the matched disturbances
% saturation status: off
% model is established by the driving force provided by the motor

%% basic parameters set of agents
Radius = [0.20,0.22,0.21,0.19,0.23,0.18];

%% assign the parameter according to serial number
serial_num = 5; 
R=Radius(serial_num);

%% current states of the robot
dimension=3;

x=agent_x(1);
y=agent_x(2);
theta=agent_x(dimension);

%% time-varying matched disturbances
% matched_disturbance= [0.5*sin(1.5*t+pi/4*serial_num+x)+2; 0.6*cos(2*t+pi/3*serial_num+0.5*y)+1.5; 0.5*sin(0.8*t+pi/5*serial_num+0.4*theta)+1];

% matched_disturbance= [0.5*sin(1.5*t+pi/4*serial_num)+2; 0.6*cos(2*t+pi/3*serial_num)+1.5; 0.5*sin(0.8*t+pi/5*serial_num)+1];
matched_disturbance = 0.2 * [0.5*sin(x) + 0.5*sin(0.6*t + pi/5*serial_num); - 0.6*exp(-abs(y)-1) + 0.4*sin(0.4*t + pi/5*serial_num) ; 0.2 * cos(theta) + 0.3 * sin(0.5*t + pi/5*serial_num)];
%% the real model of robot
g=[-sin(theta), -sin(pi/3-theta), sin(pi/3+theta);
    cos(theta), -cos(pi/3-theta), -cos(pi/3+theta);
    1/R,          1/R,                  1/R];

%% plant output
w = matched_disturbance;

v_dot = w + g* control_input;

end

== matlab function MAS_FTESO/Control and plant 1/Information subtracting ==
  data: e_xi output; L input; info_commu input; info_control input; delta_xi output; delta_vi output; a_di output; u_i_hat output; s_i output
function [e_xi, delta_xi, delta_vi, a_di, u_i_hat, s_i]=info_subtracting(L, info_commu,info_control)

%% This function is built to subtract the useful information for the controller design

% info_commu is in the format of [x_1,v_1,....,x_N,v_N]
% info_control is in the format of [delta_xi, delta_vi, a_di, w_i_hat]

serial_num = 1;
dimension = 3;
lambda = 2;

% For multiple system, we first seperate info_commu into delta_xi and delta_vi
num_agent = size(L,1);

delta_x = kron( kron(eye(num_agent) , [1,0] ), eye(dimension) ) * info_commu;
delta_v = kron( kron(eye(num_agent) , [0,1] ), eye(dimension) ) * info_commu;

L_i = kron( L(serial_num,:), eye(dimension) );
    
% Local errors calculating
e_xi = L_i * delta_x;
e_vi = L_i * delta_v;

% Substracting info_control
delta_xi = info_control(dimension*0+1:dimension*1);
delta_vi = info_control(dimension*1+1:dimension*2);

a_di = info_control(dimension*2+1:dimension*3);
u_i_hat = info_control(dimension*3+1:dimension*4);

% Slide variable
s_i = lambda * e_xi + e_vi;

end

== matlab function MAS_FTESO/Control and plant 6/MATLAB Function ==
  data: u input; y output
function y = fcn(u)

y = norm(u);

end

== matlab function MAS_FTESO/Control and plant 6/System Plant1 ==
  settings: updateMethod=DISCRETE
  data: agent_x input; v_dot output; agent_v input; t input; control_input input; w output
function [v_dot, w] = physical_model( agent_x , agent_v, t, control_input )

%% Note
% System output
% v_dot: the acceleration vector
% w: the matched disturbances
% saturation status: off
% model is established by the driving force provided by the motor

%% basic parameters set of agents
Radius = [0.20,0.22,0.21,0.19,0.23,0.18];

%% assign the parameter according to serial number
serial_num = 6; 
R=Radius(serial_num);

%% current states of the robot
dimension=3;

x=agent_x(1);
y=agent_x(2);
theta=agent_x(dimension);

%% time-varying matched disturbances
% matched_disturbance= [0.5*sin(1.5*t+pi/4*serial_num+x)+2; 0.6*cos(2*t+pi/3*serial_num+0.5*y)+1.5; 0.5*sin(0.8*t+pi/5*serial_num+0.4*theta)+1];

% matched_disturbance= [0.5*sin(1.5*t+pi/4*serial_num)+2; 0.6*cos(2*t+pi/3*serial_num)+1.5; 0.5*sin(0.8*t+pi/5*serial_num)+1];
matched_disturbance = 0.2 * [0.5*sin(x) + 0.5*sin(0.6*t + pi/5*serial_num); - 0.6*exp(-abs(y)-1) + 0.4*sin(0.4*t + pi/5*serial_num) ; 0.2 * cos(theta) + 0.3 * sin(0.5*t + pi/5*serial_num)];
%% the real model of robot
g=[-sin(theta), -sin(pi/3-theta), sin(pi/3+theta);
    cos(theta), -cos(pi/3-theta), -cos(pi/3+theta);
    1/R,          1/R,                  1/R];

%% plant output
w = matched_disturbance;

v_dot = w + g* control_input;

end

== matlab function MAS_FTESO/Self-calculation 6/Observer1/Observer iteration ==
  data: state_hat_dot output; state input; u_i input; x_tilde input; state_hat input
function state_hat_dot  = eso(state, u_i, x_tilde, state_hat)

serial_num = 6;
dimension = 3;
Radius = [0.20,0.22,0.21,0.19,0.23,0.18];
R = Radius(serial_num);
theta = state(dimension);
g=[-sin(theta), -sin(pi/3-theta), sin(pi/3+theta);
    cos(theta), -cos(pi/3-theta), -cos(pi/3+theta);
    1/R,          1/R,                  1/R];

alpha_1 = 4/5;
alpha_2 = 3/5;
beta_1 = 5 * eye(3);
beta_2 = 10 * eye(3);
beta_3 = 100 * eye(3);
rho = 2 * eye(3);

x_hat_dot = state_hat(dimension * 1 + 1 : dimension * 2) + beta_1 * (diag(sign(x_tilde)) * abs(x_tilde).^alpha_1 + x_tilde );
v_hat_dot = state_hat(dimension * 2 + 1 : dimension * 3) + beta_2 * (diag(sign(x_tilde)) * abs(x_tilde).^alpha_2 + rho * x_tilde ) + g * u_i;
w_hat_dot = beta_3 * ( diag(sign(x_tilde)) * abs(x_tilde).^alpha_2 + rho * x_tilde );

state_hat_dot = [x_hat_dot; v_hat_dot; w_hat_dot]; 

end

== matlab function MAS_FTESO/Self-calculation 2/Observer/Observer iteration ==
  data: state_hat_dot output; state input; u_i input; x_tilde input; state_hat input
function state_hat_dot  = eso(state, u_i, x_tilde, state_hat)

serial_num = 2;
dimension = 3;
Radius = [0.20,0.22,0.21,0.19,0.23,0.18];
R = Radius(serial_num);
theta = state(dimension);
g=[-sin(theta), -sin(pi/3-theta), sin(pi/3+theta);
    cos(theta), -cos(pi/3-theta), -cos(pi/3+theta);
    1/R,          1/R,                  1/R];

alpha_1 = 4/5;
alpha_2 = 3/5;
beta_1 = 5 * eye(3);
beta_2 = 10 * eye(3);
beta_3 = 100 * eye(3);
rho = 2 * eye(3);

x_hat_dot = state_hat(dimension * 1 + 1 : dimension * 2) + beta_1 * (diag(sign(x_tilde)) * abs(x_tilde).^alpha_1 + x_tilde );
v_hat_dot = state_hat(dimension * 2 + 1 : dimension * 3) + beta_2 * (diag(sign(x_tilde)) * abs(x_tilde).^alpha_2 + rho * x_tilde ) + g * u_i;
w_hat_dot = beta_3 * ( diag(sign(x_tilde)) * abs(x_tilde).^alpha_2 + rho * x_tilde );

state_hat_dot = [x_hat_dot; v_hat_dot; w_hat_dot]; 

end

== matlab function MAS_FTESO/Self-calculation 3/Tracking error calculation/Data selection ==
  data: ref input; delta_xi output; state input; delta_vi output; a_d output
function [delta_xi, delta_vi, a_d] = data_selection(ref, state)

%% This function is built to select the reference information and obtain the tracking error
serial_num = 3; 
dimension = 3;
num_agent = 6;

% Seperate the reference vector
pos_ref = ref(dimension*num_agent * 0 + 1 : dimension*num_agent * 1);
vel_ref = ref(dimension*num_agent * 1 + 1 : dimension*num_agent * 2);
acc_ref = ref(dimension*num_agent * 2 + 1 : dimension*num_agent * 3);

% Find out the reference for the current agent
pos_d = pos_ref( (serial_num-1) * dimension + 1 : serial_num * dimension);
vel_d = vel_ref( (serial_num-1) * dimension + 1 : serial_num * dimension);
acc_d = acc_ref( (serial_num-1) * dimension + 1 : serial_num * dimension);

% Seperate the state vector
x_i = state(dimension*0+1:dimension*1);
v_i = state(dimension*1+1:dimension*2);

% Calculate the error
delta_xi = x_i - pos_d;
delta_vi = v_i - vel_d;
a_d = acc_d;


end

== matlab function MAS_FTESO/Control and plant 2/Information subtracting ==
  data: e_xi output; L input; info_commu input; info_control input; delta_xi output; delta_vi output; a_di output; u_i_hat output; s_i output
function [e_xi, delta_xi, delta_vi, a_di, u_i_hat, s_i]=info_subtracting(L, info_commu,info_control)

%% This function is built to subtract the useful information for the controller design

% info_commu is in the format of [x_1,v_1,....,x_N,v_N]
% info_control is in the format of [delta_xi, delta_vi, a_di, w_i_hat]

serial_num = 2;
dimension = 3;
lambda = 2;

% For multiple system, we first seperate info_commu into delta_xi and delta_vi
num_agent = size(L,1);

delta_x = kron( kron(eye(num_agent) , [1,0] ), eye(dimension) ) * info_commu;
delta_v = kron( kron(eye(num_agent) , [0,1] ), eye(dimension) ) * info_commu;

L_i = kron( L(serial_num,:), eye(dimension) );
    
% Local errors calculating
e_xi = L_i * delta_x;
e_vi = L_i * delta_v;

% Substracting info_control
delta_xi = info_control(dimension*0+1:dimension*1);
delta_vi = info_control(dimension*1+1:dimension*2);

a_di = info_control(dimension*2+1:dimension*3);
u_i_hat = info_control(dimension*3+1:dimension*4);

% Slide variable
s_i = lambda * e_xi + e_vi;

end

== matlab function MAS_FTESO/Control and plant 2/LP-based controller/Linear programming optimisation ==
  data: u_nom input; u_i output; G_i input; now output; expect output; expect input
function [u_i, now, expect] = linear_programming(u_nom, G_i, expect)

%% This function performs the optimisation via linear programming
% Input:
% u_ei: The nominal sliding mode control input for error reduction
% u_mi: The nominal sliding mode control input for acceleration tracking
% G_i: The control gain matrix
% Output:
% u_i: The optimised control input
% expect: The expected control performance

%% Find out the constrains
U_M = 0.2;

% Saturate the maintain control input
% u_mi_max = U_M;
% u_mi = min( u_mi_max * ones(size(u_mi)) , max(u_mi , - u_mi_max * ones(size(u_mi))) );

flag = 0;
u_i = u_nom;
for i = 1 : size(u_i,1)
    if abs(u_i(i))>U_M
        flag = 1;   % flag turns 1 if the limit is reached
        break;
    end
end

% Call the linear programming solver from MATLAB
coder.extrinsic('linprog');

if flag == 1
    
    %% Intialisation
    % Restrictions on inequalities
    A_ine = zeros(2*size(u_nom,1), size(u_nom,1));
    b_ine = zeros(2*size(u_nom,1), 1);
    num_ine = 0;
    
    % Restrictions on qualities
    A_equ = zeros(2*size(u_nom,1), size(u_nom,1));
    b_equ = zeros(2*size(u_nom,1), 1);
    num_equ = 0;
    
    %% Upper and lower bound from saturation
    lb = - U_M * ones(size(u_nom));
    ub = U_M * ones(size(u_nom));
    
    %% Restrictions according to expect
    for i = 1 : size(u_nom,1)
        if expect(i) == 0 % leading to equalities
            num_equ = num_equ + 1;
            A_equ(num_equ, :) = G_i(i,:);
        else
            % No extra effort
            num_ine = num_ine + 1;
            A_ine(num_ine,:) = sign(expect(i)) * G_i(i,:);
            b_ine(num_ine) = abs(expect(i));
            
            % Avoid inverse effect (same sign)
            num_ine = num_ine + 1;
            A_ine(num_ine,:) = - sign(expect(i)) * G_i(i,:);
            
        end
    end
    
    %% Restriction to keep the same direction   
       
    % Average cost function
    F_4 = -G_i(1,:) * sign(expect(1)) - G_i(2,:) * sign(expect(2)) - G_i(3,:) * sign(expect(3));
    
    F_5 = -G_i(1,:) * expect(1) - G_i(2,:) * expect(2) - G_i(3,:) * expect(3);
    
    F=F_4;

    u_i = linprog(F,A_ine(1:num_ine,:),b_ine(1:num_ine), A_equ(1:num_equ,:), b_equ(1:num_equ),lb,ub);
end

now = G_i * u_i;

end

== matlab function MAS_FTESO/Control and plant 2/LP-based controller/Nominal Controller ==
  data: x_i input; u_i output; delta_xi input; delta_vi input; a_di input; u_i_hat input; s_i input; xi_i input; G_i output; expect output
function [u_i, G_i, expect] = fcn(x_i, delta_xi, delta_vi, a_di, u_i_hat, s_i, xi_i)

%% This is the controller design for each agent
%% Controller parameters
c_i = 2;
lambda_i = 2;

%% Basic model parameters
Radius = [0.20,0.22,0.21,0.19,0.23,0.18];   

%% The parameter of individual agent
serial_num = 2; 
R=Radius(serial_num);

%% Robot orientation
theta = x_i(3);

%% Input coupling matrix
G_i=[-sin(theta), -sin(pi/3-theta), sin(pi/3+theta);
    cos(theta), -cos(pi/3-theta), -cos(pi/3+theta);
    1/R,          1/R,                  1/R];

%% Nominal control input
expect = a_di - u_i_hat - lambda_i * delta_vi - c_i * s_i - delta_xi - c_i * xi_i;
u_i = G_i^(-1) * expect;

end

== matlab function MAS_FTESO/Control and plant 2/LP-based controller/Subsystem/Auxiliary variable ==
  data: G_i input; u_tilde input; xi_dot output; xi_prev input
function xi_dot = aux_updata(G_i, u_tilde, xi_prev)

eta_4 = diag([3,3,2]);
eta_5 = diag([0.5,0.5,0.5]);

if norm(xi_prev) >= 10
    xi_dot = eta_4 * G_i * u_tilde - eta_5 * xi_prev;
else
    xi_dot = eta_4 * G_i * u_tilde - eta_5 * xi_prev - norm(u_tilde)^2/norm(xi_prev)^2 * xi_prev;
end

end
